simulink model "Android_Battery"  (R2020a)
settings: Solver=VariableStepAuto  StartTime=0.0  StopTime=10.0  RelTol=1e-3
undefined symbols (not defined in the file): Ion, Lithium
libraries: powerlib x5, androiduilib x4, electricdrivelib x1
settings Model: Creator=kushalgoswami  LastModifiedBy=kushalgoswami

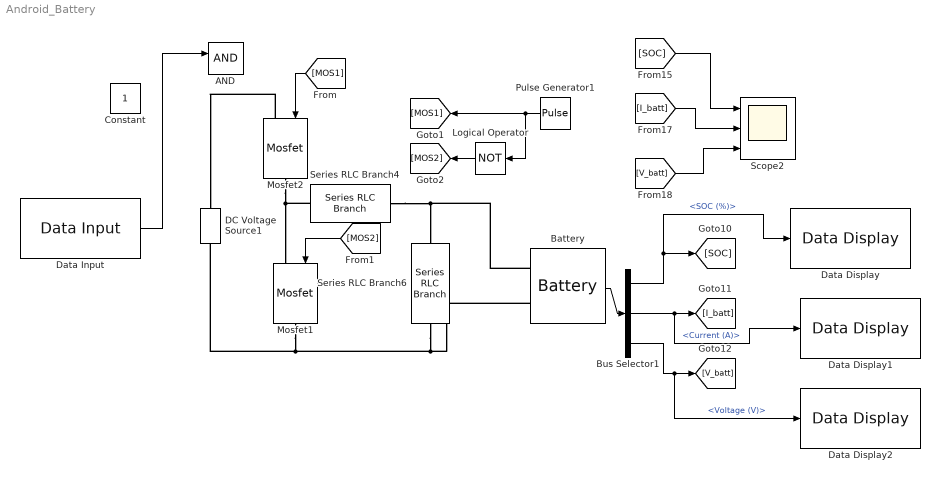
== system Android_Battery ==
  AND : Logic  IconShape=distinctive  AllPortsSameDT=off  OutDataTypeStr=boolean
  Battery : electricdrivelib/Extra Sources/Battery  BatType=Lithium-Ion  ShowTempParam=off  ThermalPreset=no  ShowAgeParam=off  NomV=24  NomQ=10  SOC=50  Batt_Tr=1e-4  PresetModel=on  MaxQ=10  MinV=18  FullV=27.9357  Dis_rate=4.3478  R=0.024  Normal_OP=9.0435  expZone="[25.9293     0.491304]"  current=[6.5 13 32.5]  Units=Time  Tci=20  NomT=20  T2=-30  MaxQ2=4.8  FullV2=7.1  Normal_OP2=5.655  expZone2="[6.58           1]"  Rca=0.6  ti=2000  Dp=0  Neq0=0  Tsim=1e6  Ta1=25  Qeol=5.4*0.9  Reol=0.013333*1.2  Char_age=[2.3478, 3]  Dis_age=[2.3478, 10]  N1=1500  N2=10500  N3=1000  N4=1400  Ta2=45  N5=950
  Bus Selector1 : BusSelector  OutputSignals=SOC (%),Current (A),Voltage (V)
  Constant : Constant
  DC Voltage Source1 : powerlib/Electrical Sources/DC Voltage Source  Amplitude=48  Measurements=None
  Data Display : androiduilib/Data Display  Format=Float  Precision=6  SimulateUsing=Code generation  blockPlatform=Android
      settings: SourceProductBaseCode=ANDROID
  Data Display1 : androiduilib/Data Display  Format=Float  Precision=6  SimulateUsing=Code generation  blockPlatform=Android
      settings: SourceProductBaseCode=ANDROID
  Data Display2 : androiduilib/Data Display  Format=Float  Precision=6  SimulateUsing=Code generation  blockPlatform=Android
      settings: SourceProductBaseCode=ANDROID
  Data Input : androiduilib/Data Input  isCharVector=off  Value=1.0  CharVector=Hello World  OutputDataType=double  maxCharVectorSize=100  SampleTime=0.1
      settings: SourceProductBaseCode=ANDROID
  Logical Operator : Logic  Operator=NOT  IconShape=distinctive  AllPortsSameDT=off  OutDataTypeStr=boolean
  Mosfet1 : powerlib/Power Electronics/Mosfet  Ron=0.1  Lon=0  Rd=0.01  Vfd=0  IC=0  Rs=1e5  Cs=inf  Measurements=off
  Mosfet2 : powerlib/Power Electronics/Mosfet  Ron=0.1  Lon=0  Rd=0.01  Vfd=0  IC=0  Rs=1e5  Cs=inf  Measurements=off
  Pulse Generator1 : DiscretePulseGenerator  PulseType=Time based  Period=1e-4  PulseWidth=60
  Scope2 : Scope  NumInputPorts=3
  Series RLC Branch4 : powerlib/Elements/Series RLC Branch  LConnTagsString=__new0  RConnTagsString=__new0  BranchType=RL  Resistance=0.05  Inductance=5.76e-2  SetiL0=off  InitialCurrent=0  Capacitance=1e-6  Setx0=off  InitialVoltage=0  Measurements=None
  Series RLC Branch6 : powerlib/Elements/Series RLC Branch  LConnTagsString=__new0  RConnTagsString=__new0  BranchType=RC  Resistance=0.001  Inductance=5.76e-4  SetiL0=off  InitialCurrent=0  Capacitance=1000e-6  Setx0=off  InitialVoltage=0  Measurements=None
  wires:
  Bus Selector1/1 -> Data Display/1, [SOC]  "<SOC (%)>"
  [MOS2] -> Mosfet1/1
  Bus Selector1/3 -> Data Display2/1, [V_batt]  "<Voltage (V)>"
  [SOC] -> Scope2/1
  [MOS1] -> Mosfet2/1
  Bus Selector1/2 -> Data Display1/1, [I_batt]  "<Current (A)>"
  Pulse Generator1/1 -> Logical Operator/1, [MOS1]
  Battery/1 -> Bus Selector1/1
  Logical Operator/1 -> [MOS2]
  [I_batt] -> Scope2/2
  [V_batt] -> Scope2/3
  Data Input/1 -> AND/1
  connections:
  DC Voltage Source1/LConn1 -- Battery/LConn2 -- Series RLC Branch6/RConn1 -- Mosfet1/RConn1
  Battery/LConn1 -- Series RLC Branch4/RConn1 -- Series RLC Branch6/LConn1
  Series RLC Branch4/LConn1 -- Mosfet2/RConn1 -- Mosfet1/LConn1
  Mosfet2/LConn1 -- DC Voltage Source1/RConn1
